simulink model "zad0"  (R2024a)
settings: Solver=VariableStepAuto  StartTime=0.0  StopTime=10.0  RelTol=1e-3
settings Model: Creator=zv53855  LastModifiedBy=zv53855

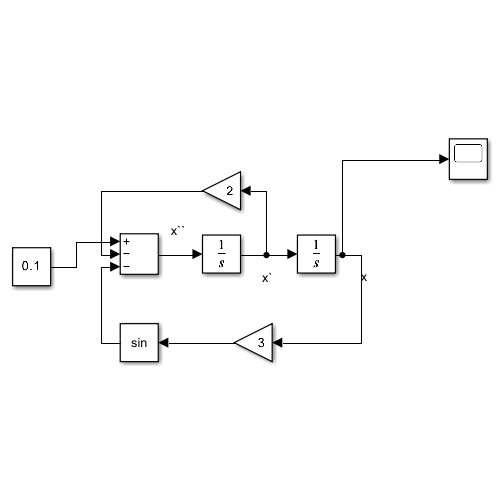
[thumbnail: Simulink's stored preview of the top-level diagram]
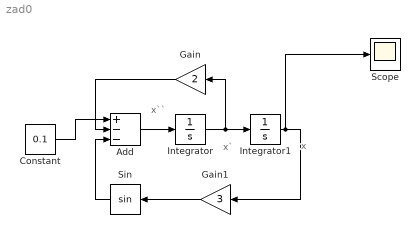
== system zad0 ==
  note: x``
  note: x`
  note: x
  Add : Sum  Inputs=+--
  Constant : Constant  Value=0.1
  Gain : Gain  Gain=2
  Gain1 : Gain  Gain=3
  Integrator : Integrator  InitialCondition=2
  Integrator1 : Integrator
  Scope : Scope
  Sin : Trigonometry
  wires:
  Integrator/1 -> Gain/1, Integrator1/1
  Add/1 -> Integrator/1
  Integrator1/1 -> Scope/1, Gain1/1
  Constant/1 -> Add/1
  Sin/1 -> Add/3
  Gain/1 -> Add/2
  Gain1/1 -> Sin/1
